simulink model "ex9"  (R2016a)
settings: Solver=VariableStepAuto  StartTime=0.0  StopTime=10.0  RelTol=1e-3
settings Model: Creator=Brand Frank  LastModifiedBy=Brand Frank

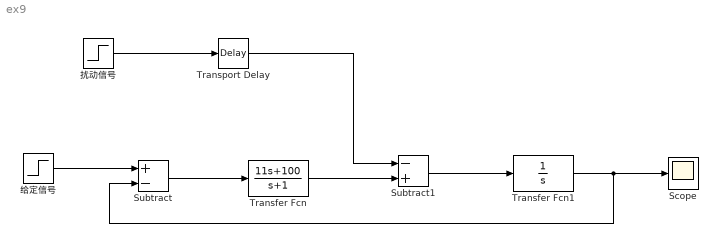
== system ex9 ==
  Scope : Scope
  Subtract : Sum  Inputs=+-
  Subtract1 : Sum  Inputs=-+
  Transfer Fcn : TransferFcn  Numerator=[11 100]  Denominator=[1 1]
  Transfer Fcn1 : TransferFcn  Denominator=[1 0]
  Transport Delay : TransportDelay  DelayTime=0.3
  扰动信号 : Step  SampleTime=0
  给定信号 : Step  SampleTime=0
  wires:
  扰动信号/1 -> Transport Delay/1
  Subtract1/1 -> Transfer Fcn1/1
  Transfer Fcn/1 -> Subtract1/2
  Transport Delay/1 -> Subtract1/1
  Transfer Fcn1/1 -> Subtract/2, Scope/1
  给定信号/1 -> Subtract/1
  Subtract/1 -> Transfer Fcn/1
